simulink model "XOO_Control"  (R2020a)
settings: Solver=FixedStepAuto  StartTime=0.0  StopTime=10.0  FixedStep=1e-3  RelTol=1e-3  EnableMultiTasking=on
settings Model: ExtModeTrigDuration=5  Creator=WinnieTrandinh  LastModifiedBy=WinnieTrandinh
settings OptimizationCC: EnhancedBackFolding=on  PassReuseOutputArgsAs=Individual arguments  ZeroExternalMemoryAtStartup=off  ZeroInternalMemoryAtStartup=off  MaxStackSize=64  OptimizeBlockOrder=speed  DifferentSizesBufferReuse=on  OptimizationCustomize=off  EfficientTunableParamExpr=on
settings DebuggingCC: ParameterTunabilityLossMsg=error
settings HardwareCC: ProdBitPerPointer=32  ProdBitPerSizeT=32  ProdBitPerPtrDiffT=32  ProdLargestAtomicInteger=Long  ProdLargestAtomicFloat=Double  ProdWordSize=32  ProdHWDeviceType=ARM Compatible->ARM Cortex
settings SFSimCC: MATLABDynamicMemAlloc=off
settings RTWCC: SystemTargetFile=ert.tlc  HardwareBoard=NXP FRDM-K64F  TemplateMakefile=ert_default_tmf  Toolchain=GNU Tools for ARM Embedded Processors
settings CodeAppCC: ForceParamTrailComments=on  IgnoreCustomStorageClasses=off  OperatorAnnotations=on  SimulinkDataObjDesc=on  SFDataObjDesc=on  InsertBlockDesc=on

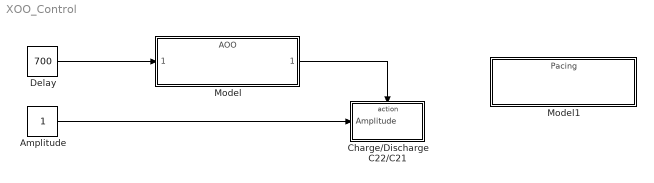
== system XOO_Control ==
  Amplitude : Constant
  Charge/Discharge C22/C21 : Subsystem  TreatAsAtomicUnit=on
  Delay : Constant  Value=700
  Model : ModelReference  ModelNameDialog=AOO.slx  SimulationMode=Normal  ModelReferenceVersion=1.5
  Model1 : ModelReference  ModelNameDialog=Pacing.slx  SimulationMode=Normal  ModelReferenceVersion=1.1
  wires:
  Delay/1 -> Model/1
  Model/1 -> Charge/Discharge C22/C21/Action
  Amplitude/1 -> Charge/Discharge C22/C21/1(Amplitude)

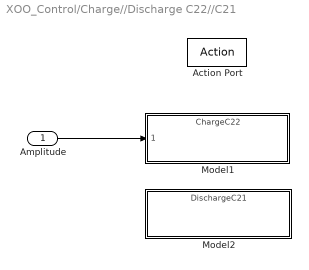
== system XOO_Control/Charge//Discharge C22//C21 ==
  Amplitude : Inport
  Action Port : ActionPort
  Model1 : ModelReference  ModelNameDialog=ChargeC22.slx  SimulationMode=Normal  ModelReferenceVersion=1.9
  Model2 : ModelReference  ModelNameDialog=DischargeC21.slx  SimulationMode=Normal  ModelReferenceVersion=1.2
  wires:
  Amplitude/1 -> Model1/1
